simulink model "FormStateBus"  (R2018b)
settings: configuration reference "RPi_DynamicsRate" (kept outside this file)
settings Model: Creator=barthal  LastModifiedBy=barthal
settings ConfigSetRef: SourceLocation=Base Workspace

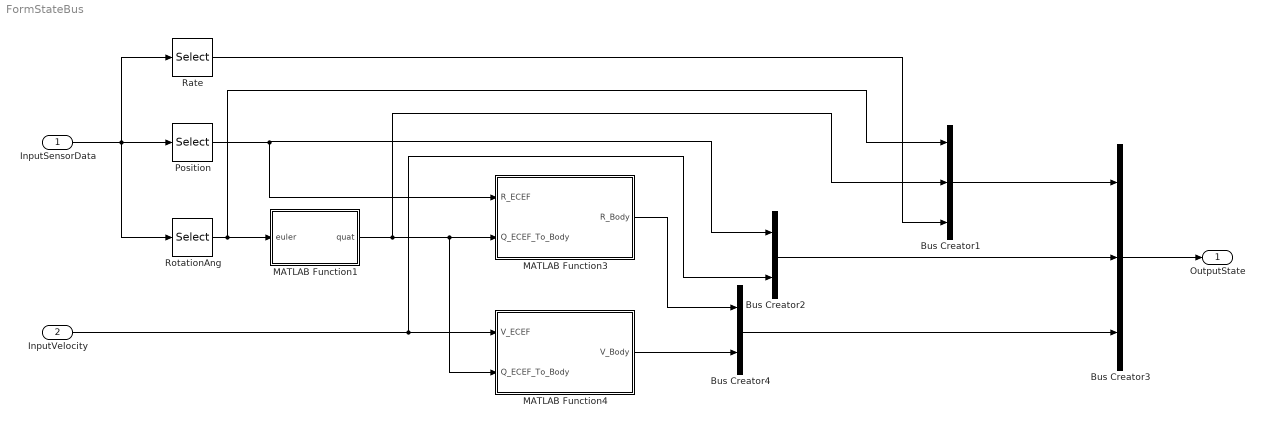
== system FormStateBus ==
  InputSensorData : Inport  PortDimensions=20
  InputVelocity : Inport  Port=2  PortDimensions=3
  Bus Creator1 : BusCreator  Inputs=3  OutDataTypeStr=Bus: RotStateBodyECEFBus
      settings: InheritFromInputs=off
  Bus Creator2 : BusCreator  Inputs=2  OutDataTypeStr=Bus: TranStateECEFBus
      settings: InheritFromInputs=off
  Bus Creator3 : BusCreator  Inputs=3  OutDataTypeStr=Bus: FullStateBus
      settings: InheritFromInputs=off
  Bus Creator4 : BusCreator  Inputs=2  OutDataTypeStr=Bus: TranStateBodyBus
      settings: InheritFromInputs=off
  MATLAB Function1 : MATLAB Function  TreatAsAtomicUnit=on
  MATLAB Function3 : MATLAB Function  TreatAsAtomicUnit=on
  MATLAB Function4 : MATLAB Function  TreatAsAtomicUnit=on
  Position : Selector  InputPortWidth=20  IndexOptions=Index vector (dialog)  Indices=[15:17]  OutputSizes=1
  Rate : Selector  InputPortWidth=20  IndexOptions=Index vector (dialog)  Indices=[4:6]  OutputSizes=1
  RotationAng : Selector  InputPortWidth=20  IndexOptions=Index vector (dialog)  Indices=[18:20]  OutputSizes=1
  OutputState : Outport  OutDataTypeStr=Bus: FullStateBus
  wires:
  RotationAng/1 -> Bus Creator1/1, MATLAB Function1/1(euler)
  Bus Creator2/1 -> Bus Creator3/2
  Bus Creator4/1 -> Bus Creator3/3
  MATLAB Function1/1(quat) -> Bus Creator1/2, MATLAB Function3/2(Q_ECEF_To_Body), MATLAB Function4/2(Q_ECEF_To_Body)
  MATLAB Function4/1(V_Body) -> Bus Creator4/2
  Rate/1 -> Bus Creator1/3
  InputVelocity/1 -> MATLAB Function4/1(V_ECEF), Bus Creator2/2
  Bus Creator3/1 -> OutputState/1
  InputSensorData/1 -> Rate/1, RotationAng/1, Position/1
  Position/1 -> Bus Creator2/1, MATLAB Function3/1(R_ECEF)
  MATLAB Function3/1(R_Body) -> Bus Creator4/1
  Bus Creator1/1 -> Bus Creator3/1

== matlab function FormStateBus/MATLAB Function1 ==
  data: quat output; euler input
function quat  = computeQuat(euler)

quat = EulerToquat_321(euler);

== matlab function FormStateBus/MATLAB Function3 ==
  data: R_Body output; R_ECEF input; Q_ECEF_To_Body input
function R_Body  = rotateVec(R_ECEF,Q_ECEF_To_Body)

R_Body = quatrotate(R_ECEF,Q_ECEF_To_Body);

== matlab function FormStateBus/MATLAB Function4 ==
  data: V_Body output; V_ECEF input; Q_ECEF_To_Body input
function V_Body  = rotateVec(V_ECEF,Q_ECEF_To_Body)

V_Body = quatrotate(V_ECEF,Q_ECEF_To_Body);
